simulink model "STATEFLOW"  (R2024b)
settings: configuration reference "STM32H7_Config" (kept outside this file)
settings Model: DataDictionary=Master_Dictionary.sldd  EnableAccessToBaseWorkspace=off  Creator=torni  LastModifiedBy=oxbro
settings ConfigSetRef: SourceName=STM32H7_Config

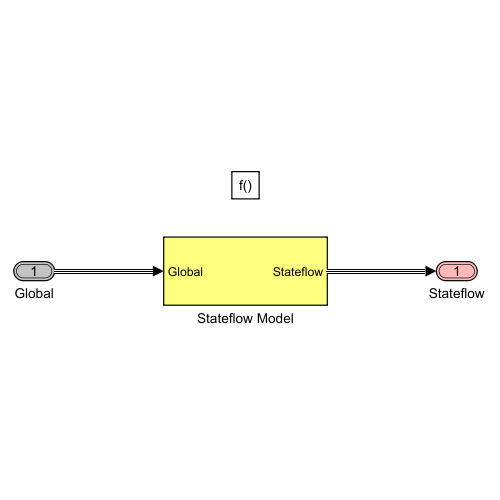
[thumbnail: Simulink's stored preview of the top-level diagram]
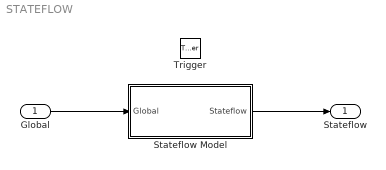
== system STATEFLOW ==
  "Global " : Inport  OutDataTypeStr=Bus: Global
  Trigger : TriggerPort  TriggerType=function-call  VariantControl=Variant  PortDimensions=1
  Stateflow Model : Subsystem
  Stateflow : Outport  OutDataTypeStr=Bus: StateflowBus  VectorParamsAs1DForOutWhenUnconnected=off
  wires:
  Stateflow Model/1(Stateflow) -> Stateflow/1
  "Global "/1 -> Stateflow Model/1(Global)

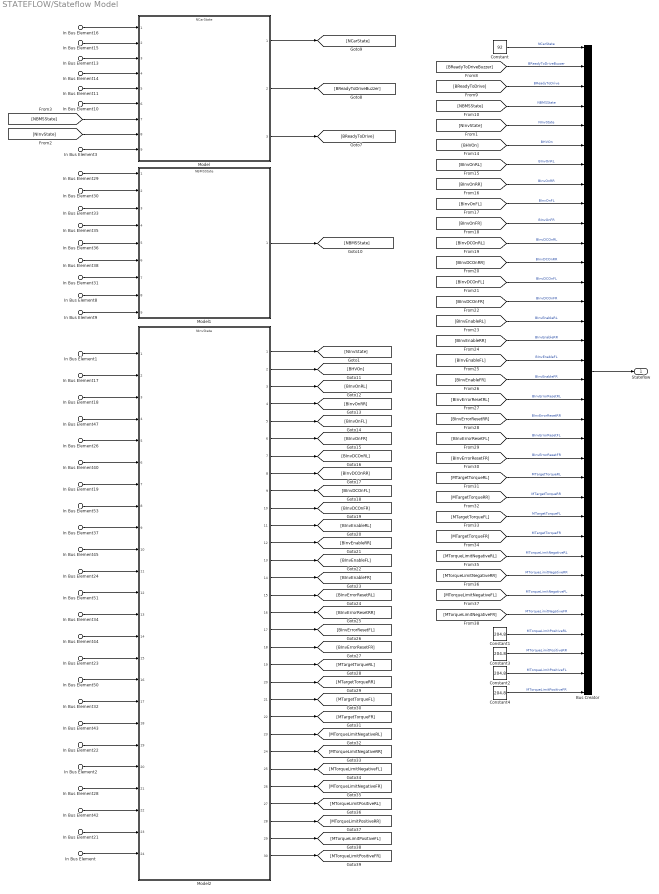
== system STATEFLOW/Stateflow Model ==
  In Bus Element29 : Inport  PortName=Global  Element=BMSSignalsBus.BBMSP0A0C
  In Bus Element30 : Inport  PortName=Global  Element=BMSSignalsBus.BBMSP0A0E
  In Bus Element33 : Inport  PortName=Global  Element=BMSSignalsBus.BBMSP0A10
  In Bus Element35 : Inport  PortName=Global  Element=BMSSignalsBus.BBMSP0A80
  In Bus Element36 : Inport  PortName=Global  Element=BMSSignalsBus.BBMSP0AC0
  In Bus Element38 : Inport  PortName=Global  Element=BMSSignalsBus.BBMSP0AFA
  In Bus Element31 : Inport  PortName=Global  Element=BMSSignalsBus.RCellAverage
  In Bus Element8 : Inport  PortName=Global  Element=BMSSignalsBus.BBalancingActive
  In Bus Element : Inport  PortName=Global  Element=BMSSignalsBus.VDCAccumulator
  In Bus Element9 : Inport  PortName=Global  Element=BMSSignalsBus.VCellAverage
  In Bus Element15 : Inport  PortName=Global  Element=SystemsBus.rThrottlePedal
  In Bus Element16 : Inport  PortName=Global  Element=SystemsBus.BErrorReset
  In Bus Element1 : Inport  PortName=Global  Element=SystemsBus.BErrorReset
  In Bus Element3 : Inport  PortName=Global  Element=SystemsBus.BReadyToDriveButton
  In Bus Element13 : Inport  PortName=Global  Element=SensorSignalsBus.pBrakeF
  In Bus Element14 : Inport  PortName=Global  Element=SensorSignalsBus.pBrakeR
  In Bus Element11 : Inport  PortName=Global  Element=InverterSignalsBus.InverterRLSignalsBus.VDCInvRL
  In Bus Element17 : Inport  PortName=Global  Element=InverterSignalsBus.InverterRLSignalsBus.VDCInvRL
  In Bus Element10 : Inport  PortName=Global  Element=InverterSignalsBus.InverterRLSignalsBus.nMotorRL
  In Bus Element18 : Inport  PortName=Global  Element=InverterSignalsBus.InverterRLSignalsBus.nMotorRL
  In Bus Element47 : Inport  PortName=Global  Element=InverterSignalsBus.InverterRLSignalsBus.BInvErrorRL
  In Bus Element50 : Inport  PortName=Global  Element=InverterSignalsBus.InverterRLSignalsBus.BInvQuitInvOnRL
  In Bus Element51 : Inport  PortName=Global  Element=InverterSignalsBus.InverterRLSignalsBus.BInvSysReadyRL
  In Bus Element53 : Inport  PortName=Global  Element=InverterSignalsBus.InverterRLSignalsBus.NInvDTCRL
  In Bus Element2 : Inport  PortName=Global  Element=InverterSignalsBus.InverterRLSignalsBus.BInvDCQuitInvOnRL
  In Bus Element40 : Inport  PortName=Global  Element=InverterSignalsBus.InverterFLSignalsBus.BInvErrorFL
  In Bus Element42 : Inport  PortName=Global  Element=InverterSignalsBus.InverterFLSignalsBus.BInvDCQuitInvOnFL
  In Bus Element43 : Inport  PortName=Global  Element=InverterSignalsBus.InverterFLSignalsBus.BInvQuitInvOnFL
  In Bus Element44 : Inport  PortName=Global  Element=InverterSignalsBus.InverterFLSignalsBus.BInvSysReadyFL
  In Bus Element45 : Inport  PortName=Global  Element=InverterSignalsBus.InverterFLSignalsBus.NInvDTCFL
  In Bus Element26 : Inport  PortName=Global  Element=InverterSignalsBus.InverterRRSignalsBus.BInvErrorRR
  In Bus Element28 : Inport  PortName=Global  Element=InverterSignalsBus.InverterRRSignalsBus.BInvDCQuitInvOnRR
  In Bus Element32 : Inport  PortName=Global  Element=InverterSignalsBus.InverterRRSignalsBus.BInvQuitInvOnRR
  In Bus Element34 : Inport  PortName=Global  Element=InverterSignalsBus.InverterRRSignalsBus.BInvSysReadyRR
  In Bus Element37 : Inport  PortName=Global  Element=InverterSignalsBus.InverterRRSignalsBus.NInvDTCRR
  In Bus Element19 : Inport  PortName=Global  Element=InverterSignalsBus.InverterFRSignalsBus.BInvErrorFR
  In Bus Element21 : Inport  PortName=Global  Element=InverterSignalsBus.InverterFRSignalsBus.BInvDCQuitInvOnFR
  In Bus Element22 : Inport  PortName=Global  Element=InverterSignalsBus.InverterFRSignalsBus.BInvQuitInvOnFR
  In Bus Element23 : Inport  PortName=Global  Element=InverterSignalsBus.InverterFRSignalsBus.BInvSysReadyFR
  In Bus Element24 : Inport  PortName=Global  Element=InverterSignalsBus.InverterFRSignalsBus.NInvDTCFR
  Bus Creator : BusCreator  Inputs=34  OutDataTypeStr=Bus: StateflowBus
  Constant : Constant  Value=92
  Constant{1..4} (4 alike) : Constant  Value=204.8
  Model : ModelReference  ModelNameDialog=NCarState.slx  SimulationMode=Normal  ModelReferenceVersion=13.5
  Model1 : ModelReference  ModelNameDialog=NBMSState.slx  SimulationMode=Normal  ModelReferenceVersion=13.5
  Model2 : ModelReference  ModelNameDialog=NInvState.slx  SimulationMode=Normal  ModelReferenceVersion=13.6
  Stateflow : Outport  OutDataTypeStr=Bus: StateflowBus  VectorParamsAs1DForOutWhenUnconnected=off
  wires:
  Model1/1 -> [NBMSState]
  In Bus Element29/1 -> Model1/1
  In Bus Element38/1 -> Model1/6
  In Bus Element35/1 -> Model1/4
  In Bus Element33/1 -> Model1/3
  In Bus Element30/1 -> Model1/2
  In Bus Element36/1 -> Model1/5
  Bus Creator/1 -> Stateflow/1
  In Bus Element31/1 -> Model1/7
  In Bus Element8/1 -> Model1/8
  In Bus Element15/1 -> Model/2
  In Bus Element13/1 -> Model/3
  In Bus Element14/1 -> Model/4
  In Bus Element11/1 -> Model/5
  [NInvState] -> Model/8
  Model/1 -> [NCarState]
  Model/2 -> [BReadyToDriveBuzzer]
  Model/3 -> [BReadyToDrive]
  In Bus Element9/1 -> Model1/9
  [NInvState] -> Bus Creator/5  "NInvState"
  [BInvOnRL] -> Bus Creator/7  "BInvOnRL"
  [BInvOnRR] -> Bus Creator/8  "BInvOnRR"
  [BInvOnFL] -> Bus Creator/9  "BInvOnFL"
  [BInvOnFR] -> Bus Creator/10  "BInvOnFR"
  [BInvDCOnRL] -> Bus Creator/11  "BInvDCOnRL"
  [BInvDCOnRR] -> Bus Creator/12  "BInvDCOnRR"
  [BInvDCOnFL] -> Bus Creator/13  "BInvDCOnFL"
  [BInvDCOnFR] -> Bus Creator/14  "BInvDCOnFR"
  [BInvEnableRL] -> Bus Creator/15  "BInvEnableRL"
  In Bus Element1/1 -> Model2/1
  In Bus Element17/1 -> Model2/2
  In Bus Element18/1 -> Model2/3
  In Bus Element47/1 -> Model2/4
  In Bus Element26/1 -> Model2/5
  In Bus Element40/1 -> Model2/6
  In Bus Element19/1 -> Model2/7
  In Bus Element53/1 -> Model2/8
  In Bus Element37/1 -> Model2/9
  In Bus Element45/1 -> Model2/10
  In Bus Element24/1 -> Model2/11
  In Bus Element51/1 -> Model2/12
  In Bus Element34/1 -> Model2/13
  In Bus Element44/1 -> Model2/14
  In Bus Element23/1 -> Model2/15
  In Bus Element32/1 -> Model2/17
  In Bus Element43/1 -> Model2/18
  In Bus Element22/1 -> Model2/19
  In Bus Element50/1 -> Model2/16
  In Bus Element28/1 -> Model2/21
  In Bus Element42/1 -> Model2/22
  In Bus Element21/1 -> Model2/23
  Model2/1 -> [NInvState]
  Model2/2 -> [BHVOn]
  Model2/3 -> [BInvOnRL]
  Model2/4 -> [BInvOnRR]
  Model2/5 -> [BInvOnFL]
  Model2/6 -> [BInvOnFR]
  Model2/7 -> [BInvDCOnRL]
  Model2/8 -> [BInvDCOnRR]
  Model2/9 -> [BInvDCOnFL]
  Model2/10 -> [BInvDCOnFR]
  Model2/11 -> [BInvEnableRL]
  Model2/12 -> [BInvEnableRR]
  Model2/13 -> [BInvEnableFL]
  Model2/14 -> [BInvEnableFR]
  Model2/15 -> [BInvErrorResetRL]
  Model2/16 -> [BInvErrorResetRR]
  Model2/17 -> [BInvErrorResetFL]
  Model2/18 -> [BInvErrorResetFR]
  Model2/19 -> [MTargetTorqueRL]
  Model2/20 -> [MTargetTorqueRR]
  Model2/21 -> [MTargetTorqueFL]
  Model2/22 -> [MTargetTorqueFR]
  Model2/23 -> [MTorqueLimitNegativeRL]
  Model2/24 -> [MTorqueLimitNegativeRR]
  Model2/25 -> [MTorqueLimitNegativeFL]
  Model2/26 -> [MTorqueLimitNegativeFR]
  Model2/27 -> [MTorqueLimitPositiveRL]
  Model2/28 -> [MTorqueLimitPositiveRR]
  Model2/29 -> [MTorqueLimitPositiveFL]
  Model2/30 -> [MTorqueLimitPositiveFR]
  [BHVOn] -> Bus Creator/6  "BHVOn"
  [BInvEnableRR] -> Bus Creator/16  "BInvEnableRR"
  [BInvEnableFL] -> Bus Creator/17  "BInvEnableFL"
  [BInvEnableFR] -> Bus Creator/18  "BInvEnableFR"
  [BInvErrorResetRL] -> Bus Creator/19  "BInvErrorResetRL"
  [BInvErrorResetRR] -> Bus Creator/20  "BInvErrorResetRR"
  [BInvErrorResetFL] -> Bus Creator/21  "BInvErrorResetFL"
  [BInvErrorResetFR] -> Bus Creator/22  "BInvErrorResetFR"
  [MTargetTorqueRL] -> Bus Creator/23  "MTargetTorqueRL"
  [MTargetTorqueRR] -> Bus Creator/24  "MTargetTorqueRR"
  [MTargetTorqueFL] -> Bus Creator/25  "MTargetTorqueFL"
  [MTargetTorqueFR] -> Bus Creator/26  "MTargetTorqueFR"
  [MTorqueLimitNegativeRL] -> Bus Creator/27  "MTorqueLimitNegativeRL"
  [MTorqueLimitNegativeRR] -> Bus Creator/28  "MTorqueLimitNegativeRR"
  [MTorqueLimitNegativeFL] -> Bus Creator/29  "MTorqueLimitNegativeFL"
  [MTorqueLimitNegativeFR] -> Bus Creator/30  "MTorqueLimitNegativeFR"
  Constant1/1 -> Bus Creator/31  "MTorqueLimitPositiveRL"
  Constant3/1 -> Bus Creator/32  "MTorqueLimitPositiveRR"
  Constant2/1 -> Bus Creator/33  "MTorqueLimitPositiveFL"
  Constant4/1 -> Bus Creator/34  "MTorqueLimitPositiveFR"
  In Bus Element/1 -> Model2/24
  In Bus Element10/1 -> Model/6
  In Bus Element2/1 -> Model2/20
  [NBMSState] -> Model/7
  In Bus Element16/1 -> Model/1
  In Bus Element3/1 -> Model/9
  [NBMSState] -> Bus Creator/4  "NBMSState"
  [BReadyToDrive] -> Bus Creator/3  "BReadyToDrive"
  [BReadyToDriveBuzzer] -> Bus Creator/2  "BReadyToDriveBuzzer"
  Constant/1 -> Bus Creator/1  "NCarState"
